simulink model "Solar_Array_with_Boost_Converter_with_PO_MPPT_4kW"  (R2024a)
settings: Solver=VariableStepAuto  StartTime=0.0  StopTime=3  RelTol=1e-3
libraries: spsSeriesRLCBranchLib x4, spsCurrentMeasurementLib x1, spsDiodeLib x1, spsIGBTDiodeLib x1, spsPVArrayLib x1, spsPWMGeneratorDCDCLib x1, spsVoltageMeasurementLib x1, sps_lib x1
settings Model: Creator=KimoStore  LastModifiedBy=KimoStore

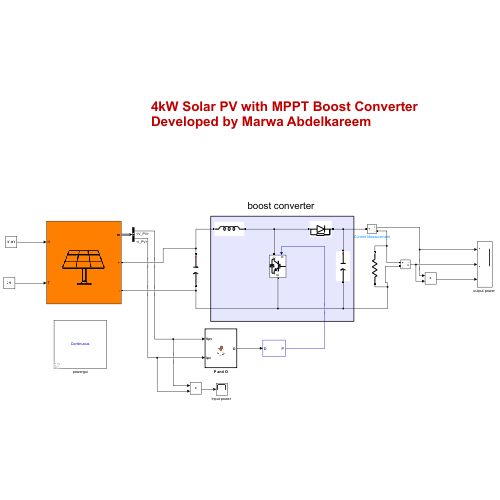
[thumbnail: Simulink's stored preview of the top-level diagram]
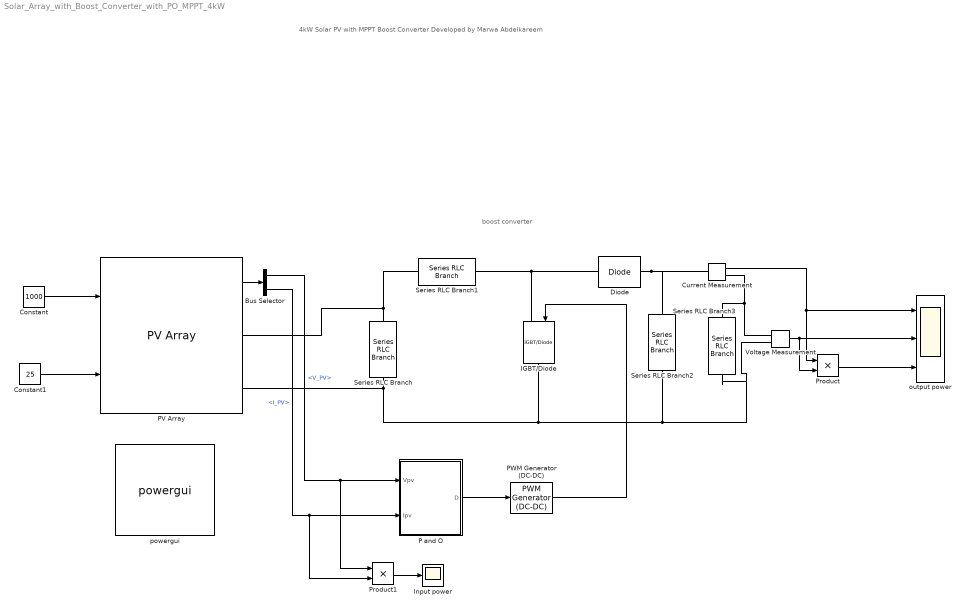
== system Solar_Array_with_Boost_Converter_with_PO_MPPT_4kW ==
  note: boost converter
  note: 4kW Solar PV with MPPT Boost Converter
      | Developed by Marwa Abdelkareem
  Bus Selector : BusSelector  OutputSignals=V_PV,I_PV
  Constant : Constant  Value=1000
  Constant1 : Constant  Value=25
  Current Measurement : spsCurrentMeasurementLib/Current Measurement  PhasorSimulation=off  OutputType=Complex  PSBequivalent=0
  Diode : spsDiodeLib/Diode  Ron=0.001  Lon=0  Vf=0.8  IC=0  UseSnubber=0  Rs=500  Cs=250e-9  Measurements=off
  IGBT/Diode : spsIGBTDiodeLib/IGBT//Diode  Ron=1e-3  Rs=1e5  Cs=inf  Measurements=off
  "Input power " : Scope
  P and O : MATLAB Function  TreatAsAtomicUnit=on
  PV Array : spsPVArrayLib/PV Array  Npar=4  Nser=4  PlotType=array @ 25 deg.C & specified irradiances  S_vec="[ 1000  500  100 ]"  Temp_C_vec="[ 45 25  ]"  ModuleName=User-defined  PlotWhenSelected=off  Pm=250.205  Ncell=60  Voc=37.3  Isc=8.66  Vm=30.7  Im=8.15  beta_Voc_pc=-0.36901  alpha_Isc_pc=0.086998  beta_Voc=-0.13764  alpha_Isc=0.007534  IL=8.7062  I0=4.1579e-10  nI=1.0189  Rsh=240.6015  Rs=0.23732  RobustModel=off  RobustCellTemperature=25  BAL=on  Tc=1e-6  Tfilter=5e-5
  PWM Generator (DC-DC) : spsPWMGeneratorDCDCLib/PWM Generator (DC-DC)  Fsw=5e3  Ts=0
  Product : Product
  Product1 : Product
  Series RLC Branch : spsSeriesRLCBranchLib/Series RLC Branch  LConnTagsString=__new0  RConnTagsString=__new0  BranchType=C  Resistance=1  Inductance=1e-3  SetiL0=off  InitialCurrent=0  Capacitance=0.001283715555556  Setx0=off  InitialVoltage=0  Measurements=None
  Series RLC Branch1 : spsSeriesRLCBranchLib/Series RLC Branch  LConnTagsString=__new0  RConnTagsString=__new0  BranchType=L  Resistance=1  Inductance=0.018215048725290  SetiL0=off  InitialCurrent=0  Capacitance=1e-6  Setx0=off  InitialVoltage=0  Measurements=None
  Series RLC Branch2 : spsSeriesRLCBranchLib/Series RLC Branch  LConnTagsString=__new0  RConnTagsString=__new0  BranchType=C  Resistance=1  Inductance=1e-3  SetiL0=off  InitialCurrent=0  Capacitance=0.001283715555556  Setx0=off  InitialVoltage=0  Measurements=None
  Series RLC Branch3 : spsSeriesRLCBranchLib/Series RLC Branch  LConnTagsString=__new0  RConnTagsString=__new0  BranchType=R  Resistance=9.202453987730062  Inductance=1e-3  SetiL0=off  InitialCurrent=0  Capacitance=1e-6  Setx0=off  InitialVoltage=0  Measurements=None
  Voltage Measurement : spsVoltageMeasurementLib/Voltage Measurement  PhasorSimulation=off  OutputType=Complex  PSBequivalent=0
  "output power " : Scope  NumInputPorts=3
  powergui : sps_lib/powergui  Priority=1  SimulationMode=Continuous  SampleTime=50e-6  frequency=60  Iterations=50  frequencyindice=0  Pbase=100e6  ErrMax=1e-4  UnitsV=kV  UnitsW=MW  buscounter=0  FunctionMessages=off  echomessages=off  EnableUseOfTLC=off  CurrentSourceSwitches=off  DisableSnubberDevices=off  DisableRonSwitches=off  DisableVfSwitches=off  DisplayEquations=off  AutomaticDiscreteSolvers=off  SolverType=Tustin/Backward Euler (TBE)  Interpol=off  ExternalGateDelay=off  methode=off  Ts=100  x0status=blocks  SPID=on  SwTol=0  HookPort=off  NonlinearTolerance=1e-4  nMaxIteration=100  ContinueOnMaxIteration=off  RestoreLinks=warning  ResistiveCurrentMeasurement=off  Frange=[0:2:500]  Ylog=off  Xlog=on  ShowGrid=off  save=off  variable=ZData  structure=0  ZoomFFT=off  StartTime=0.0  cycles=1  DisplayStyle=1  fundamental=60  FreqAxis=off  MaxFrequency=1000  frequencyindicesteady=1  RmsSteady=1  display=off
  wires:
  Voltage Measurement/1 -> Product/2, "output power "/2
  Constant/1 -> PV Array/1
  Product1/1 -> "Input power "/1
  Constant1/1 -> PV Array/2
  PWM Generator (DC-DC)/1 -> IGBT/Diode/1
  Bus Selector/1 -> Product1/1, P and O/1(Vpv)  "<V_PV>"
  Product/1 -> "output power "/3
  PV Array/1 -> Bus Selector/1
  Bus Selector/2 -> Product1/2, P and O/2(Ipv)  "<I_PV>"
  Current Measurement/1 -> "output power "/1, Product/1
  P and O/1(D) -> PWM Generator (DC-DC)/1
  connections:
  IGBT/Diode/LConn1 -- Diode/LConn1 -- Series RLC Branch1/RConn1
  Series RLC Branch/LConn1 -- PV Array/RConn1 -- Series RLC Branch1/LConn1
  Diode/RConn1 -- Current Measurement/LConn1 -- Series RLC Branch2/LConn1
  Voltage Measurement/LConn1 -- Series RLC Branch3/LConn1 -- Current Measurement/RConn1
  IGBT/Diode/RConn1 -- Series RLC Branch3/RConn1 -- Voltage Measurement/LConn2 -- Series RLC Branch2/RConn1 -- PV Array/RConn2 -- Series RLC Branch/RConn1

== matlab function Solar_Array_with_Boost_Converter_with_PO_MPPT_4kW/P and O ==
  settings: updateMethod=DISCRETE  sampleTime=1e-4
  data: Vpv input; D output; Ipv input
function D = P_O(Vpv,Ipv)
 Dmax=0.9;
 Dmin=0.1;
 Dinit=0.9;
 deltaD=1e-4;
 persistent Dpre Ppre Vpre;
 
 %first run
     if isempty(Dpre)
         Dpre=Dinit;
         Vpre=0;
         Ppre=0;
     end
 Ppv=Vpv*Ipv;
 dp=Ppv-Ppre;
 dv=Vpv-Vpre;
 
     if dp~=0 
             if(dp>0)
                     if(dv<0)
                         D=Dpre+deltaD;
                     else
                         D=Dpre-deltaD;
                     end     
             else                   
                     if(dv<0)
                         D=Dpre-deltaD;
                     else
                         D=Dpre+deltaD;
                     end
             end   
    else
          D=Dpre;
    end
    
    if D>=Dmax || D <= Dmin
        D=Dpre;
    end
    
    Ppre=Ppv;
    Vpre=Vpv;
    Dpre=D;
end
